simulink model "sstv_transmit"  (R2022a)
settings: Solver=FixedStepAuto  StartTime=0.0  StopTime=120  FixedStep=0.1  RelTol=1e-3
model workspace (MAT data in the model file):
  components = reshape([0 0 0 0 0 0 0 0 0 0 0 0 0 0 0 0 0 0 0 0 0 0 2 2 2 0 0 1 1 0 0 0 0 0 0 0 0 0 0 0 2 2 0 0 0 1 1 0 0 1 1 1 1 1 1 1 1 1 1 1 0 0 3 3 3 0 0 0 0 2 2 2 2 2 2 2 2 0 0 0 3 3 0 0 0 0 0 0 0 3 3 3 3 3 3 3 3 2 2 2 0 0 0 0 0 2 2 0 0 4 4 4 4 4 4 4 0 0 0 0 1 1 1 1 1 0 0 0 0 0 0 0 0 0 0 0 0 3 3 3 0 0 0 0 0 0 0 0 0 0 0 0 0 0 0 0 0 0 0 0 0 0 0 0 0 0 3 0 0 0 0 0 0 0 0 0 0 0 0 0 0 0 0 0 0 0 0 0 0 0 0 0 0 0 0 0 0 0 0 0 0 0 2 2 2 0 0 1 1 0 0 0 0 0 0 0 0 0 0 0 2 2 0 0 0 1 1 0 0 1 1 1 1 1 1 1 1 1 1 1 0 0 3 3 3 0 0 0 0 2 2 2 2 2 2 2 2 0 0 0 3 3 0 0 0 0 0 0 0 3 3 3 3 3 3 3 3 2 2 2 0 0 0 0 0 3 2 0 0 4 4 4 4 4 4 4 0 0 0 0 1 1 1 1 1 0 0 0 0 0 0 0 0 0 0 0 0 3 3 3 0 0 0 0 0 0 0 0 0 0 0 0 0 0 0 0 0 0 0 0 0 0 0 0 0 0 3 0 0 0 0 0 0 0 0 0 0 0 0 0], [20 9 2])
  counts = [8; 8; 7; 7; 7; 6; 9; 2; 2; 6; 6; 6; 6; 6; 6; 6; 5; 8; 8; 8]
  durations = [0.004862 0.004862 0.0015 0.0015 0.0015 0.009 0.009 0.007 0.007 0.02 0.02 0.02 ... (360 elements, 20x9x2)]
  modeTable = [44  320  256  256  1  0  0  0; 40  320  256  256  1  0  0  0; 60  320  256  256  1  0.009  0  0; 56  320  256  256  1  0.009  0  0; 76  320  256  256  1  0.009  0  0; 8  320  240  240  1  0  1  1; 12  320  240  240  1  0  1  0; 2  160  120  120  1  0  1  0; 6  160  120  120  1  0  1  0; 93  320  256  128  2  0  1  1; 99  320  256  128  2  0  1  1; 95  640  496  248  2  0  1  1; 98  512  400  200  2  0  1  1; 96  640  496  248  2  0  1  1; 97  640  496  248  2  0  1  1; 94  800  616  308  2  0  1  1; 55  320  256  256  1  0  0  0; 113  640  496  496  1  0  0  0; 114  640  496  496  1  0  0  0; 115  640  496  496  1  0  0  0]
  tones = reshape([1200 1200 1500 1500 1500 1200 1200 1200 1200 1200 1200 1200 1200 1200 1200 1200 1200 1200 1200 1200 1500 1500 0 0 0 1500 1500 0 0 1500 1500 1500 1500 1500 1500 1500 1500 1500 1500 1500 0 0 1500 1500 1500 0 0 0 0 0 0 0 0 0 0 0 0 0 0 0 1500 1500 0 0 0 1500 1500 0 0 0 0 0 0 0 0 0 0 1500 1500 1500 0 0 1200 1200 1200 1900 1900 0 0 0 0 0 0 0 0 0 0 0 0 0 1500 1500 1500 1500 1500 0 0 0 0 0 0 0 0 0 0 0 0 1500 1500 1500 0 0 0 0 0 0 2300 0 0 0 0 0 0 0 0 0 0 0 0 0 1500 1500 0 0 0 0 1500 0 0 0 0 0 0 0 0 0 0 1500 1500 1500 0 0 0 0 0 0 0 0 0 0 0 0 0 0 0 0 0 0 0 0 1200 1200 1500 1500 1500 1200 1200 1200 1200 1200 1200 1200 1200 1200 1200 1200 1200 1200 1200 1200 1500 1500 0 0 0 1500 1500 0 0 1500 1500 1500 1500 1500 1500 1500 1500 1500 1500 1500 0 0 1500 1500 1500 0 0 0 0 0 0 0 0 0 0 0 0 0 0 0 1500 1500 0 0 0 2300 1500 0 0 0 0 0 0 0 0 0 0 1500 1500 1500 0 0 1200 1200 1200 1900 1900 0 0 0 0 0 0 0 0 0 0 0 0 0 1500 1500 1500 1500 1500 0 0 0 0 0 0 0 0 0 0 0 0 1500 1500 1500 0 0 0 0 0 0 2300 0 0 0 0 0 0 0 0 0 0 0 0 0 1500 1500 0 0 0 0 1500 0 0 0 0 0 0 0 0 0 0 1500 1500 1500 0 0 0 0 0 0 0 0 0 0 0 0 0 0 0 0 0 0 0 0], [20 9 2])
settings Model: DataDictionary=sstv_transmit.sldd  Creator=luoch  LastModifiedBy=luoch
settings DataIOCC: SaveOutput=off  SignalLogging=off
settings ModelReferenceCC: EnableRefExpFcnMdlSchedulingChecks=off
settings RTWCC: Description=Generic Real-Time Target  GPUComputeCapability=5.0
settings ConfigComp: CovBoundaryAbsTol=1.0e-5

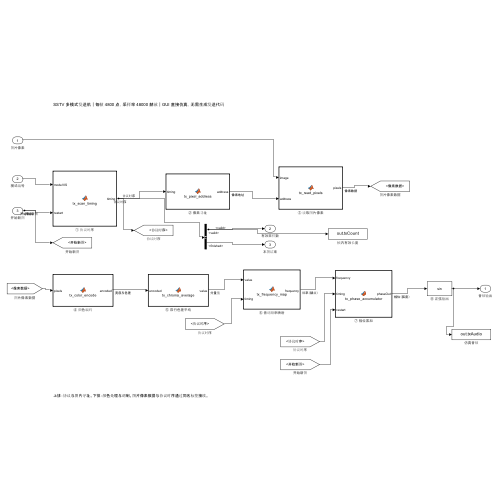
[thumbnail: Simulink's stored preview of the top-level diagram]
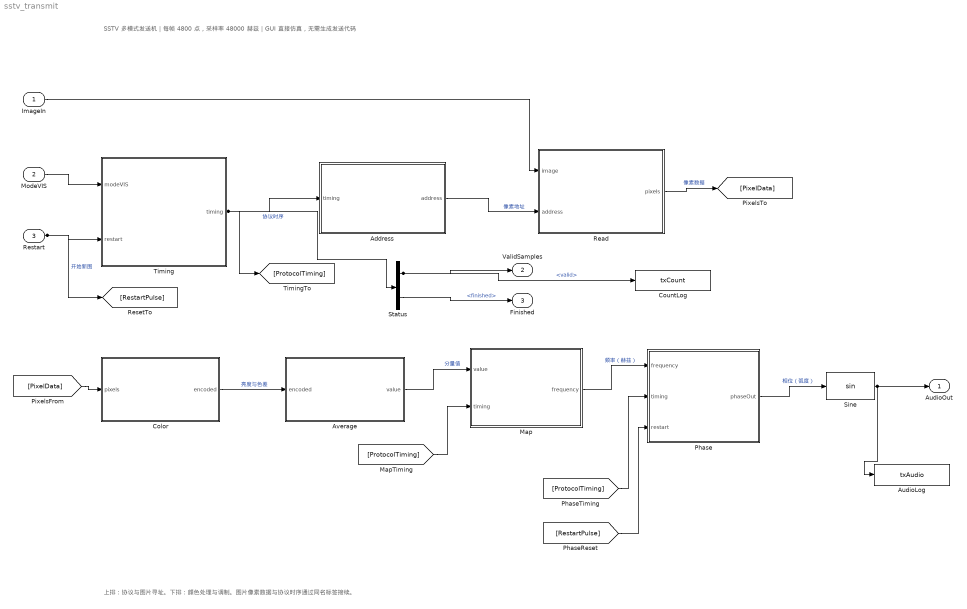
== system sstv_transmit ==
  note: SSTV 多模式发送机｜每帧 4800 点，采样率 48000 赫兹｜GUI 直接仿真，无需生成发送代码
  note: 上排：协议与图片寻址。下排：颜色处理与调制。图片像素数据与协议时序通过同名标签接续。
  ImageIn : Inport  OutDataTypeStr=uint8  PortDimensions=1478400  SampleTime=0.1
      settings: AttributesFormatString=图片像素
  ModeVIS : Inport  Port=2  OutDataTypeStr=uint8  PortDimensions=1  SampleTime=0.1
      settings: AttributesFormatString=模式编号
  Restart : Inport  Port=3  OutDataTypeStr=boolean  PortDimensions=1  SampleTime=0.1
      settings: AttributesFormatString=开始新图
  Address : MATLAB Function  TreatAsAtomicUnit=on
      settings: AttributesFormatString=② 像素寻址
  AudioLog : ToWorkspace  VariableName=txAudio  SampleTime=-1
      settings: AttributesFormatString=仿真音频
  Average : MATLAB Function  TreatAsAtomicUnit=on
      settings: AttributesFormatString=⑤ 双行色差平均
  Color : MATLAB Function  TreatAsAtomicUnit=on
      settings: AttributesFormatString=④ 颜色编码
  CountLog : ToWorkspace  VariableName=txCount  SampleTime=-1
      settings: AttributesFormatString=帧内有效长度
  Map : MATLAB Function  TreatAsAtomicUnit=on
      settings: AttributesFormatString=⑥ 音调频率映射
  Phase : MATLAB Function  TreatAsAtomicUnit=on
      settings: AttributesFormatString=⑦ 相位累加
  Read : MATLAB Function  TreatAsAtomicUnit=on
      settings: AttributesFormatString=③ 读取图片像素
  Sine : Trigonometry
      settings: AttributesFormatString=⑧ 正弦输出
  Status : BusSelector  OutputSignals=valid,finished
  Timing : MATLAB Function  TreatAsAtomicUnit=on
      settings: AttributesFormatString=① 协议时序
  AudioOut : Outport
      settings: AttributesFormatString=音频输出
  ValidSamples : Outport  Port=2
      settings: AttributesFormatString=有效采样数
  Finished : Outport  Port=3
      settings: AttributesFormatString=本图结束
  wires:
  ModeVIS/1 -> Timing/1(modeVIS)
  Restart/1 -> Timing/2(restart), [RestartPulse]  "开始新图"
  Timing/1(timing) -> Address/1(timing), [ProtocolTiming], Status/1  "协议时序"
  ImageIn/1 -> Read/1(image)
  Address/1(address) -> Read/2(address)  "像素地址"
  Color/1(encoded) -> Average/1(encoded)  "亮度与色差"
  Average/1(value) -> Map/1(value)  "分量值"
  Map/1(frequency) -> Phase/1(frequency)  "频率（赫兹）"
  Phase/1(phaseOut) -> Sine/1  "相位（弧度）"
  Read/1(pixels) -> [PixelData]  "像素数据"
  [PixelData] -> Color/1(pixels)
  [ProtocolTiming] -> Map/2(timing)
  [ProtocolTiming] -> Phase/2(timing)
  [RestartPulse] -> Phase/3(restart)
  Sine/1 -> AudioOut/1, AudioLog/1
  Status/1 -> ValidSamples/1, CountLog/1  "<valid>"
  Status/2 -> Finished/1  "<finished>"

== matlab function sstv_transmit/Address ==
  data: timing input; address output Bus: sstvTxAddress
function address=tx_pixel_address(timing)
%#codegen
% 扫描行组和段内时间转换为像素地址；双行模式另给出共享色差的伙伴行。
address=struct('row',zeros(4800,1,'uint16'),'column',zeros(4800,1,'uint16'), ...
    'other',zeros(4800,1,'uint16'),'component',timing.component,'color',timing.color,'pair',timing.pair);
for k=1:4800
    if timing.component(k)==0,continue,end
    row=(double(timing.unit(k))-1)*timing.rowsPerUnit+1;
    if timing.component(k)==4,row=row+1;address.component(k)=uint8(1);end
    address.row(k)=uint16(row);
    address.column(k)=uint16(max(1,min(timing.width,1+floor(timing.elapsed(k)/(timing.duration(k)/timing.width)))));
    other=2*floor((row-1)/2)+1;if other==row,other=other+1;end
    address.other(k)=uint16(other);
end
end

== matlab function sstv_transmit/Timing ==
  data: modeVIS input; timing output Bus: sstvTxTiming; restart input; modeTable parameter; durations parameter; components parameter; tones parameter; counts parameter
function timing = tx_scan_timing(modeVIS,restart,modeTable, durations, components, tones, counts)
%#codegen
% 逐采样生成 VIS、行同步及像素地址。累计时间确定边界，状态跨处理帧保留。
% 模式表列：VIS、宽、高、行组数、每组行数、起始同步秒数、颜色类型、共享色差。
persistent sample elapsed duration boundary stage segment unit modeIndex channel hz done
if isempty(sample) || restart
    sample=0;elapsed=0;duration=.3;boundary=14400;stage=0;segment=1;unit=1;
    modeIndex=1;channel=0;hz=1900;done=true;
    for m=1:20
        if modeTable(m,1)==double(modeVIS),modeIndex=m;done=false;break,end
    end
end
timing=struct('unit',zeros(4800,1,'uint16'),'elapsed',zeros(4800,1),'duration',zeros(4800,1), ...
    'component',zeros(4800,1,'uint8'),'tone',zeros(4800,1),'valid',uint16(0),'finished',false, ...
    'width',modeTable(modeIndex,2),'rowsPerUnit',modeTable(modeIndex,5), ...
    'color',uint8(modeTable(modeIndex,7)),'pair',logical(modeTable(modeIndex,8)));
for k=1:4800
    if done,break,end
    if sample>=boundary
        elapsed=elapsed+duration;
        if stage==0
            segment=segment+1;
            if segment>13
                segment=1;
                if modeTable(modeIndex,6)>0,stage=1;else,stage=2;end
            end
        elseif stage==1
            stage=2;segment=1;
        elseif stage==2
            segment=segment+1;
            if segment>counts(modeIndex)
                segment=1;unit=unit+1;
                if unit>modeTable(modeIndex,4),stage=3;end
            end
        else
            done=true;break
        end
        channel=0;
        if stage==0
            duration=.03;hz=1200;
            if segment==2,duration=.01;
            elseif segment==3,duration=.3;hz=1900;
            elseif segment>=5 && segment<=11
                hz=1300-200*double(bitget(modeVIS,segment-4));
            elseif segment==12
                onesCount=0;for bit=1:7,onesCount=onesCount+double(bitget(modeVIS,bit));end
                hz=1300-200*mod(onesCount,2);
            end
        elseif stage==1
            duration=modeTable(modeIndex,6);hz=1200;
        elseif stage==2
            variant=1+mod(unit-1,2);
            duration=durations(modeIndex,segment,variant);
            channel=components(modeIndex,segment,variant);hz=tones(modeIndex,segment,variant);
        else
            duration=.1;hz=1500;
        end
        boundary=round((elapsed+duration)*48000);
    end
    timing.component(k)=uint8(channel);timing.tone(k)=hz;
    if channel>0
        timing.unit(k)=uint16(unit);
        timing.elapsed(k)=sample/48000-elapsed;timing.duration(k)=duration;
    end
    timing.valid=timing.valid+1;sample=sample+1;
end
% 最后一个有效样本恰好位于帧尾时，也在本帧给出结束标记。
timing.finished=done || (stage==3 && sample>=boundary);
end

== matlab function sstv_transmit/Read ==
  data: image input; pixels output Bus: sstvTxPixels; address input
function pixels=tx_read_pixels(image,address)
%#codegen
% 读取当前像素和伙伴行同列像素。图片以 616×800×3 列优先数组存储。
pixels=struct('rgb',zeros(4800,3),'otherRGB',zeros(4800,3), ...
    'component',address.component,'color',address.color,'pair',address.pair);
for k=1:4800
    if address.component(k)==0,continue,end
    for ch=1:3
        base=616*(double(address.column(k))-1)+616*800*(ch-1);
        pixels.rgb(k,ch)=double(image(base+double(address.row(k))));
        if address.pair
            pixels.otherRGB(k,ch)=double(image(base+double(address.other(k))));
        end
    end
end
end

== matlab function sstv_transmit/Color ==
  data: pixels input; encoded output Bus: sstvTxEncoded
function encoded=tx_color_encode(pixels)
%#codegen
% 选择 RGB 分量，或按全范围亮度/色差公式编码；限幅后再交给双行平均。
encoded=struct('value',zeros(4800,1),'other',zeros(4800,1),'average',false(4800,1));
for k=1:4800
    ch=double(pixels.component(k));if ch==0,continue,end
    if pixels.color==0
        encoded.value(k)=pixels.rgb(k,ch);
    else
        encoded.value(k)=color(pixels.rgb(k,:),ch);
        encoded.average(k)=pixels.pair && ch>1;
        if encoded.average(k),encoded.other(k)=color(pixels.otherRGB(k,:),ch);end
    end
end
end
function value=color(rgb,ch)
y=.299*rgb(1)+.587*rgb(2)+.114*rgb(3);
if ch==1,value=y;
elseif ch==2,value=128+(rgb(1)-y)/1.402;
else,value=128+(rgb(3)-y)/1.772;
end
value=max(0,min(255,value));
end

== matlab function sstv_transmit/Average ==
  data: encoded input; value output
function value=tx_chroma_average(encoded)
%#codegen
% 仅 Robot 36 与 PD 的色差共享两行，亮度及其他模式直接通过。
value=encoded.value;
for k=1:4800
    if encoded.average(k),value(k)=(value(k)+encoded.other(k))/2;end
end
end

== matlab function sstv_transmit/Map ==
  data: value input; frequency output; timing input
function frequency=tx_frequency_map(value,timing)
%#codegen
% 图像分量映射到 1500～2300 赫兹；VIS、同步与间隔采用协议指定音调。
frequency=timing.tone;
for k=1:4800
    if timing.component(k)>0,frequency(k)=1500+800*value(k)/255;end
end
end

== matlab function sstv_transmit/Phase ==
  data: frequency input; phaseOut output; timing input; restart input
function phaseOut=tx_phase_accumulator(frequency,timing,restart)
%#codegen
% 频率积分为相位；像素、颜色分量与处理帧之间均保持相位连续。
persistent phase
if isempty(phase) || restart,phase=0;end
phaseOut=zeros(4800,1);
for k=1:double(timing.valid)
    phaseOut(k)=phase;
    phase=phase+2*pi*frequency(k)/48000;
    if phase>=2*pi,phase=phase-2*pi;end
end
end
